simulink model "MainPlanevsRainCameras"  (R2020a)
(part 3 of 6)

  Radar3 : drivingscenarioandsensors/Radar Detection Generator  SensorIndex=5  UpdateInterval=0.1  SensorLocation=[0 0.9]  Height=0.2  Yaw=170.804327895794  Pitch=0  Roll=0  BusNameSource=Auto  BusName=BusRadarDetectionGenerator  MaxNumDetectionsSource=Property  MaxNumDetections=50  DetectionCoordinates=Ego Cartesian  SimulateUsing=Interpreted execution  AzimuthResolution=4  ElevationResolution=10  RangeResolution=2.5  RangeRateResolution=0.5  AzimuthBiasFraction=0.1  ElevationBiasFraction=0.1  RangeBiasFraction=0.05  RangeRateBiasFraction=0.05  FieldOfView=[90 2.5]  MaxRange=10  RangeRateLimits=[-100 100]  DetectionProbability=0.9  FalseAlarmRate=1e-06  ReferenceRange=15  ReferenceRCS=0  HasElevation=on  HasRangeRate=off  HasNoise=on  HasFalseAlarms=on  HasOcclusion=on  InitialSeedSource=Repeatable  InitialSeed=0  UsedSeed=0  ActorProfilesSource=MATLAB expression  ActorProfilesParameters=driving.internal.ActorProfilesRadarParameters  ActorProfilesExpression=[struct('ActorID',1,'ClassID',1,'Length',4.7,'Width',1.8,'Height',1.4,'OriginOffset',[-1.35 0 0],'MeshVertices',[3.7 -0.9 1.4;3.7 0.9 1.4;-1 0.9 1.4;-1 -0.9 1.4;3.7 -0.9 0;3.7 0.9 0;-1 0.9 0;-1 -0.9 0],'MeshFaces',[6 2 1;1 5 6;8 4 3;3 7 8;6 7 3;3 2 6;5 1 4;4 8 5;4 1 2;2 3 4;7 6 5;5 8 7],'RCSPattern',[10 10;10 10],'RCSAzimuthAngles',[-180 180],'RCSElevationAngles',[-90 90]); struct('ActorID',2,'ClassID',1,'Length',4.7,'Width',1.8,'Height',1.4,'OriginOffset',[-1.35 0 0],'MeshVertices',[3.7 -0.9 1.4;3.7 0.9 1.4;-1 0.9 1.4;-1 -0.9 1.4;3.7 -0.9 0;3.7 0.9 0;-1 0.9 0;-1 -0.9 0],'MeshFaces',[6 2 1;1 5 6;8 4 3;3 7 8;6 7 3;3 2 6;5 1 4;4 8 5;4 1 2;2 3 4;7 6 5;5 8 7],'RCSPattern',[10 10;10 10],'RCSAzimuthAngles',[-180 180],'RCSElevationAngles',[-90 90]); struct('ActorID',3,'ClassID',1,'Length',4.7,'Width',1.8,'Height',1.4,'OriginOffset',[-1.35 0 0],'MeshVertices',[3.7 -0.9 1.4;3.7 0.9 1.4;-1 0.9 1.4;-1 -0.9 1.4;3.7 -0.9 0;3.7 0.9 0;-1 0.9 0;-1 -0.9 0],'MeshFaces',[6 2 1;1 5 6;8 4 3;3 7 8;6 7 3;3 2 6;5 1 4;4 8 5;4 1 2;2 3 4;7 6 5;5 8 7],'RCSPattern',[10 10;10 10],'RCSAzimuthAngles',[-180 180],'RCSElevationAngles',[-90 90]); struct('ActorID',4,'ClassID',1,'Length',4.7,'Width',1.8,'Height',1.4,'OriginOffset',[-1.35 0 0],'MeshVertices',[3.7 -0.9 1.4;3.7 0.9 1.4;-1 0.9 1.4;-1 -0.9 1.4;3.7 -0.9 0;3.7 0.9 0;-1 0.9 0;-1 -0.9 0],'MeshFaces',[6 2 1;1 5 6;8 4 3;3 7 8;6 7 3;3 2 6;5 1 4;4 8 5;4 1 2;2 3 4;7 6 5;5 8 7],'RCSPattern',[10 10;10 10],'RCSAzimuthAngles',[-180 180],'RCSElevationAngles',[-90 90]); struct('ActorID',5,'ClassID',1,'Length',4.7,'Width',1.8,'Height',1.4,'OriginOffset',[-1.35 0 0],'MeshVertices',[3.7 -0.9 1.4;3.7 0.9 1.4;-1 0.9 1.4;-1 -0.9 1.4;3.7 -0.9 0;3.7 0.9 0;-1 0.9 0;-1 -0.9 0],'MeshFaces',[6 2 1;1 5 6;8 4 3;3 7 8;6 7 3;3 2 6;5 1 4;4 8 5;4 1 2;2 3 4;7 6 5;5 8 7],'RCSPattern',[10 10;10 10],'RCSAzimuthAngles',[-180 180],'RCSElevationAngles',[-90 90]); struct('ActorID',6,'ClassID',4,'Length',0.24,'Width',0.45,'Height',1.7,'OriginOffset',[0 0 0],'MeshVertices',[0.12 -0.225 1.7;0.12 0.225 1.7;-0.12 0.225 1.7;-0.12 -0.225 1.7;0.12 -0.225 -1.11022302462516e-16;0.12 0.225 -1.11022302462516e-16;-0.12 0.225 -1.11022302462516e-16;-0.12 -0.225 -1.11022302462516e-16],'MeshFaces',[6 2 1;1 5 6;8 4 3;3 7 8;6 7 3;3 2 6;5 1 4;4 8 5;4 1 2;2 3 4;7 6 5;5 8 7],'RCSPattern',[-8 -8;-8 -8],'RCSAzimuthAngles',[-180 180],'RCSElevationAngles',[-90 90]); struct('ActorID',7,'ClassID',4,'Length',0.24,'Width',0.45,'Height',1.7,'OriginOffset',[0 0 0],'MeshVertices',[0.12 -0.225 1.7;0.12 0.225 1.7;-0.12 0.225 1.7;-0.12 -0.225 1.7;0.12 -0.225 -1.11022302462516e-16;0.12 0.225 -1.11022302462516e-16;-0.12 0.225 -1.11022302462516e-16;-0.12 -0.225 -1.11022302462516e-16],'MeshFaces',[6 2 1;1 5 6;8 4 3;3 7 8;6 7 3;3 2 6;5 1 4;4 8 5;4 1 2;2 3 4;7 6 5;5 8 7],'RCSPattern',[-8 -8;-8 -8],'RCSAzimuthAngles',[-180 180],'RCSElevationAngles',[-90 90]); struct('ActorID',8,'ClassID',4,'Length',0.24,'Width',0.45,'Height',1.7,'OriginOffset',[0 0 0],'MeshVertices',[0.12 -0.225 1.7;0.12 0.225 1.7;-0.12 0.225 1.7;-0.12 -0.225 1.7;0.12 -0.225 -1.11022302462516e-16;0.12 0.225 -1.11022302462516e-16;-0.12 0.225 -1.11022302462516e-16;-0.12 -0.225 -1.11022302462516e-16],'MeshFaces',[6 2 1;1 5 6;8 4 3;3 7 8;6 7 3;3 2 6;5 1 4;4 8 5;4 1 2;2 3 4;7 6 5;5 8 7],'RCSPattern',[-8 -8;-8 -8],'RCSAzimuthAngles',[-180 180],'RCSElevationAngles',[-90 90]); struct('ActorID',9,'ClassID',4,'Length',0.24,'Width',0.45,'Height',1.7,'OriginOffset',[0 0 0],'MeshVertices',[0.12 -0.225 1.7;0.12 0.225 1.7;-0.12 0.225 1.7;-0.12 -0.225 1.7;0.12 -0.225 -1.11022302462516e-16;0.12 0.225 -1.11022302462516e-16;-0.12 0.225 -1.11022302462516e-16;-0.12 -0.225 -1.11022302462516e-16],'MeshFaces',[6 2 1;1 5 6;8 4 3;3 7 8;6 7 3;3 2 6;5 1 4;4 8 5;4 1 2;2 3 4;7 6 5;5 8 7],'RCSPattern',[-8 -8;-8 -8],'RCSAzimuthAngles',[-180 180],'RCSElevationAngles',[-90 90]); struct('ActorID',10,'ClassID',4,'Length',0.24,'Width',0.45,'Height',1.7,'OriginOffset',[0 0 0],'MeshVertices',[0.12 -0.225 1.7;0.12 0.225 1.7;-0.12 0.225 1.7;-0.12 -0.225 1.7;0.12 -0.225 -1.11022302462516e-16;0.12 0.225 -1.11022302462516e-16;-0.12 0.225 -1.11022302462516e-16;-0.12 -0.225 -1.11022302462516e-16],'MeshFaces',[6 2 1;1 5 6;8 4 3;3 7 8;6 7 3;3 2 6;5 1 4;4 8 5;4 1 2;2 3 4;7 6 5;5 8 7],'RCSPattern',[-8 -8;-8 -8],'RCSAzimuthAngles',[-180 180],'RCSElevationAngles',[-90 90]); struct('ActorID',11,'ClassID',4,'Length',0.24,'Width',0.45,'Height',1.7,'OriginOffset',[0 0 0],'MeshVertices',[0.12 -0.225 1.7;0.12 0.225 1.7;-0.12 0.225 1.7;-0.12 -0.225 1.7;0.12 -0.225 -1.11022302462516e-16;0.12 0.225 -1.11022302462516e-16;-0.12 0.225 -1.11022302462516e-16;-0.12 -0.225 -1.11022302462516e-16],'MeshFaces',[6 2 1;1 5 6;8 4 3;3 7 8;6 7 3;3 2 6;5 1 4;4 8 5;4 1 2;2 3 4;7 6 5;5 8 7],'RCSPattern',[-8 -8;-8 -8],'RCSAzimuthAngles',[-180 180],'RCSElevationAngles',[-90 90]); struct('ActorID',12,'ClassID',4,'Length',0.24,'Width',0.45,'Height',1.7,'OriginOffset',[0 0 0],'MeshVertices',[0.12 -0.225 1.7;0.12 0.225 1.7;-0.12 0.225 1.7;-0.12 -0.225 1.7;0.12 -0.225 -1.11022302462516e-16;0.12 0.225 -1.11022302462516e-16;-0.12 0.225 -1.11022302462516e-16;-0.12 -0.225 -1.11022302462516e-16],'MeshFaces',[6 2 1;1 5 6;8 4 3;3 7 8;6 7 3;3 2 6;5 1 4;4 8 5;4 1 2;2 3 4;7 6 5;5 8 7],'RCSPattern',[-8 -8;-8 -8],'RCSAzimuthAngles',[-180 180],'RCSElevationAngles',[-90 90]); struct('ActorID',13,'ClassID',4,'Length',0.24,'Width',0.45,'Height',1.7,'OriginOffset',[0 0 0],'MeshVertices',[0.12 -0.225 1.7;0.12 0.225 1.7;-0.12 0.225 1.7;-0.12 -0.225 1.7;0.12 -0.225 -1.11022302462516e-16;0.12 0.225 -1.11022302462516e-16;-0.12 0.225 -1.11022302462516e-16;-0.12 -0.225 -1.11022302462516e-16],'MeshFaces',[6 2 1;1 5 6;8 4 3;3 7 8;6 7 3;3 2 6;5 1 4;4 8 5;4 1 2;2 3 4;7 6 5;5 8 7],'RCSPattern',[-8 -8;-8 -8],'RCSAzimuthAngles',[-180 180],'RCSElevationAngles',[-90 90]); struct('ActorID',14,'ClassID',4,'Length',0.24,'Width',0.45,'Height',1.7,'OriginOffset',[0 0 0],'MeshVertices',[0.12 -0.225 1.7;0.12 0.225 1.7;-0.12 0.225 1.7;-0.12 -0.225 1.7;0.12 -0.225 -1.11022302462516e-16;0.12 0.225 -1.11022302462516e-16;-0.12 0.225 -1.11022302462516e-16;-0.12 -0.225 -1.11022302462516e-16],'MeshFaces',[6 2 1;1 5 6;8 4 3;3 7 8;6 7 3;3 2 6;5 1 4;4 8 5;4 1 2;2 3 4;7 6 5;5 8 7],'RCSPattern',[-8 -8;-8 -8],'RCSAzimuthAngles',[-180 180],'RCSElevationAngles',[-90 90]); struct('ActorID',15,'ClassID',4,'Length',0.24,'Width',0.45,'Height',1.7,'OriginOffset',[0 0 0],'MeshVertices',[0.12 -0.225 1.7;0.12 0.225 1.7;-0.12 0.225 1.7;-0.12 -0.225 1.7;0.12 -0.225 -1.11022302462516e-16;0.12 0.225 -1.11022302462516e-16;-0.12 0.225 -1.11022302462516e-16;-0.12 -0.225 -1.11022302462516e-16],'MeshFaces',[6 2 1;1 5 6;8 4 3;3 7 8;6 7 3;3 2 6;5 1 4;4 8 5;4 1 2;2 3 4;7 6 5;5 8 7],'RCSPattern',[-8 -8;-8 -8],'RCSAzimuthAngles',[-180 180],'RCSElevationAngles',[-90 90]); struct('ActorID',16,'ClassID',4,'Length',0.24,'Width',0.45,'Height',1.7,'OriginOffset',[0 0 0],'MeshVertices',[0.12 -0.225 1.7;0.12 0.225 1.7;-0.12 0.225 1.7;-0.12 -0.225 1.7;0.12 -0.225 -1.11022302462516e-16;0.12 0.225 -1.11022302462516e-16;-0.12 0.225 -1.11022302462516e-16;-0.12 -0.225 -1.11022302462516e-16],'MeshFaces',[6 2 1;1 5 6;8 4 3;3 7 8;6 7 3;3 2 6;5 1 4;4 8 5;4 1 2;2 3 4;7 6 5;5 8 7],'RCSPattern',[-8 -8;-8 -8],'RCSAzimuthAngles',[-180 180],'RCSElevationAngles',[-90 90]); struct('ActorID',17,'ClassID',4,'Length',0.24,'Width',0.45,'Height',1.7,'OriginOffset',[0 0 0],'MeshVertices',[0.12 -0.225 1.7;0.12 0.225 1.7;-0.12 0.225 1.7;-0.12 -0.225 1.7;0.12 -0.225 -1.11022302462516e-16;0.12 0.225 -1.11022302462516e-16;-0.12 0.225 -1.11022302462516e-16;-0.12 -0.225 -1.11022302462516e-16],'MeshFaces',[6 2 1;1 5 6;8 4 3;3 7 8;6 7 3;3 2 6;5 1 4;4 8 5;4 1 2;2 3 4;7 6 5;5 8 7],'RCSPattern',[-8 -8;-8 -8],'RCSAzimuthAngles',[-180 180],'RCSElevationAngles',[-90 90]); struct('ActorID',18,'ClassID',4,'Length',0.24,'Width',0.45,'Height',1.7,'OriginOffset',[0 0 0],'MeshVertices',[0.12 -0.225 1.7;0.12 0.225 1.7;-0.12 0.225 1.7;-0.12 -0.225 1.7;0.12 -0.225 -1.11022302462516e-16;0.12 0.225 -1.11022302462516e-16;-0.12 0.225 -1.11022302462516e-16;-0.12 -0.225 -1.11022302462516e-16],'MeshFaces',[6 2 1;1 5 6;8 4 3;3 7 8;6 7 3;3 2 6;5 1 4;4 8 5;4 1 2;2 3 4;7 6 5;5 8 7],'RCSPattern',[-8 -8;-8 -8],'RCSAzimuthAngles',[-180 180],'RCSElevationAngles',[-90 90]); struct('ActorID',19,'ClassID',4,'Length',0.24,'Width',0.45,'Height',1.7,'OriginOffset',[0 0 0],'MeshVertices',[0.12 -0.225 1.7;0.12 0.225 1.7;-0.12 0.225 1.7;-0.12 -0.225 1.7;0.12 -0.225 -1.11022302462516e-16;0.12 0.225 -1.11022302462516e-16;-0.12 0.225 -1.11022302462516e-16;-0.12 -0.225 -1.11022302462516e-16],'MeshFaces',[6 2 1;1 5 6;8 4 3;3 7 8;6 7 3;3 2 6;5 1 4;4 8 5;4 1 2;2 3 4;7 6 5;5 8 7],'RCSPattern',[-8 -8;-8 -8],'RCSAzimuthAngles',[-180 180],'RCSElevationAngles',[-90 90]); struct('ActorID',20,'ClassID',4,'Length',0.24,'Width',0.45,'Height',1.7,'OriginOffset',[0 0 0],'MeshVertices',[0.12 -0.225 1.7;0.12 0.225 1.7;-0.12 0.225 1.7;-0.12 -0.225 1.7;0.12 -0.225 -1.11022302462516e-16;0.12 0.225 -1.11022302462516e-16;-0.12 0.225 -1.11022302462516e-16;-0.12 -0.225 -1.11022302462516e-16],'MeshFaces',[6 2 1;1 5 6;8 4 3;3 7 8;6 7 3;3 2 6;5 1 4;4 8 5;4 1 2;2 3 4;7 6 5;5 8 7],'RCSPattern',[-8 -8;-8 -8],'RCSAzimuthAngles',[-180 180],'RCSElevationAngles',[-90 90]); struct('ActorID',21,'ClassID',4,'Length',0.24,'Width',0.45,'Height',1.7,'OriginOffset',[0 0 0],'MeshVertices',[0.12 -0.225 1.7;0.12 0.225 1.7;-0.12 0.225 1.7;-0.12 -0.225 1.7;0.12 -0.225 -1.11022302462516e-16;0.12 0.225 -1.11022302462516e-16;-0.12 0.225 -1.11022302462516e-16;-0.12 -0.225 -1.11022302462516e-16],'MeshFaces',[6 2 1;1 5 6;8 4 3;3 7 8;6 7 3;3 2 6;5 1 4;4 8 5;4 1 2;2 3 4;7 6 5;5 8 7],'RCSPattern',[-8 -8;-8 -8],'RCSAzimuthAngles',[-180 180],'RCSElevationAngles',[-90 90]); struct('ActorID',22,'ClassID',4,'Length',0.24,'Width',0.45,'Height',1.7,'OriginOffset',[0 0 0],'MeshVertices',[0.12 -0.225 1.7;0.12 0.225 1.7;-0.12 0.225 1.7;-0.12 -0.225 1.7;0.12 -0.225 -1.11022302462516e-16;0.12 0.225 -1.11022302462516e-16;-0.12 0.225 -1.11022302462516e-16;-0.12 -0.225 -1.11022302462516e-16],'MeshFaces',[6 2 1;1 5 6;8 4 3;3 7 8;6 7 3;3 2 6;5 1 4;4 8 5;4 1 2;2 3 4;7 6 5;5 8 7],'RCSPattern',[-8 -8;-8 -8],'RCSAzimuthAngles',[-180 180],'RCSElevationAngles',[-90 90]); struct('ActorID',23,'ClassID',4,'Length',0.24,'Width',0.45,'Height',1.7,'OriginOffset',[0 0 0],'MeshVertices',[0.12 -0.225 1.7;0.12 0.225 1.7;-0.12 0.225 1.7;-0.12 -0.225 1.7;0.12 -0.225 -1.11022302462516e-16;0.12 0.225 -1.11022302462516e-16;-0.12 0.225 -1.11022302462516e-16;-0.12 -0.225 -1.11022302462516e-16],'MeshFaces',[6 2 1;1 5 6;8 4 3;3 7 8;6 7 3;3 2 6;5 1 4;4 8 5;4 1 2;2 3 4;7 6 5;5 8 7],'RCSPattern',[-8 -8;-8 -8],'RCSAzimuthAngles',[-180 180],'RCSElevationAngles',[-90 90]); struct('ActorID',24,'ClassID',4,'Length',0.24,'Width',0.45,'Height',1.7,'OriginOffset',[0 0 0],'MeshVertices',[0.12 -0.225 1.7;0.12 0.225 1.7;-0.12 0.225 1.7;-0.12 -0.225 1.7;0.12 -0.225 -1.11022302462516e-16;0.12 0.225 -1.11022302462516e-16;-0.12 0.225 -1.11022302462516e-16;-0.12 -0.225 -1.11022302462516e-16],'MeshFaces',[6 2 1;1 5 6;8 4 3;3 7 8;6 7 3;3 2 6;5 1 4;4 8 5;4 1 2;2 3 4;7 6 5;5 8 7],'RCSPattern',[-8 -8;-8 -8],'RCSAzimuthAngles',[-180 180],'RCSElevationAngles',[-90 90]); struct('ActorID',25,'ClassID',4,'Length',0.24,'Width',0.45,'Height',1.7,'OriginOffset',[0 0 0],'MeshVertices',[0.12 -0.225 1.7;0.12 0.225 1.7;-0.12 0.225 1.7;-0.12 -0.225 1.7;0.12 -0.225 -1.11022302462516e-16;0.12 0.225 -1.11022302462516e-16;-0.12 0.225 -1.11022302462516e-16;-0.12 -0.225 -1.11022302462516e-16],'MeshFaces',[6 2 1;1 5 6;8 4 3;3 7 8;6 7 3;3 2 6;5 1 4;4 8 5;4 1 2;2 3 4;7 6 5;5 8 7],'RCSPattern',[-8 -8;-8 -8],'RCSAzimuthAngles',[-180 180],'RCSElevationAngles',[-90 90]); struct('ActorID',26,'ClassID',4,'Length',0.24,'Width',0.45,'Height',1.7,'OriginOffset',[0 0 0],'MeshVertices',[0.12 -0.225 1.7;0.12 0.225 1.7;-0.12 0.225 1.7;-0.12 -0.225 1.7;0.12 -0.225 -1.11022302462516e-16;0.12 0.225 -1.11022302462516e-16;-0.12 0.225 -1.11022302462516e-16;-0.12 -0.225 -1.11022302462516e-16],'MeshFaces',[6 2 1;1 5 6;8 4 3;3 7 8;6 7 3;3 2 6;5 1 4;4 8 5;4 1 2;2 3 4;7 6 5;5 8 7],'RCSPattern',[-8 -8;-8 -8],'RCSAzimuthAngles',[-180 180],'RCSElevationAngles',[-90 90]); struct('ActorID',27,'ClassID',4,'Length',0.24,'Width',0.45,'Height',1.7,'OriginOffset',[0 0 0],'MeshVertices',[0.12 -0.225 1.7;0.12 0.225 1.7;-0.12 0.225 1.7;-0.12 -0.225 1.7;0.12 -0.225 -1.11022302462516e-16;0.12 0.225 -1.11022302462516e-16;-0.12 0.225 -1.11022302462516e-16;-0.12 -0.225 -1.11022302462516e-16],'MeshFaces',[6 2 1;1 5 6;8 4 3;3 7 8;6 7 3;3 2 6;5 1 4;4 8 5;4 1 2;2 3 4;7 6 5;5 8 7],'RCSPattern',[-8 -8;-8 -8],'RCSAzimuthAngles',[-180 180],'RCSElevationAngles',[-90 90]); struct('ActorID',28,'ClassID',3,'Length',1.7,'Width',0.45,'Height',1.7,'OriginOffset',[0 0 0],'MeshVertices',[0.85 -0.225 1.7;0.85 0.225 1.7;-0.85 0.225 1.7;-0.85 -0.225 1.7;0.85 -0.225 -1.11022302462516e-16;0.85 0.225 -1.11022302462516e-16;-0.85 0.225 -1.11022302462516e-16;-0.85 -0.225 -1.11022302462516e-16],'MeshFaces',[6 2 1;1 5 6;8 4 3;3 7 8;6 7 3;3 2 6;5 1 4;4 8 5;4 1 2;2 3 4;7 6 5;5 8 7],'RCSPattern',[10 10;10 10],'RCSAzimuthAngles',[-180 180],'RCSElevationAngles',[-90 90]); struct('ActorID',29,'ClassID',4,'Length',0.24,'Width',0.45,'Height',1.7,'OriginOffset',[0 0 0],'MeshVertices',[0.12 -0.225 1.7;0.12 0.225 1.7;-0.12 0.225 1.7;-0.12 -0.225 1.7;0.12 -0.225 -1.11022302462516e-16;0.12 0.225 -1.11022302462516e-16;-0.12 0.225 -1.11022302462516e-16;-0.12 -0.225 -1.11022302462516e-16],'MeshFaces',[6 2 1;1 5 6;8 4 3;3 7 8;6 7 3;3 2 6;5 1 4;4 8 5;4 1 2;2 3 4;7 6 5;5 8 7],'RCSPattern',[-8 -8;-8 -8],'RCSAzimuthAngles',[-180 180],'RCSElevationAngles',[-90 90])]
      settings: SourceProductBaseCode=DR
  Radar4 : drivingscenarioandsensors/Radar Detection Generator  SensorIndex=6  UpdateInterval=0.1  SensorLocation=[0 -0.9]  Height=0.2  Yaw=-171.21089543369  Pitch=0  Roll=0  BusNameSource=Auto  BusName=BusRadarDetectionGenerator  MaxNumDetectionsSource=Property  MaxNumDetections=50  DetectionCoordinates=Ego Cartesian  SimulateUsing=Interpreted execution  AzimuthResolution=4  ElevationResolution=10  RangeResolution=2.5  RangeRateResolution=0.5  AzimuthBiasFraction=0.1  ElevationBiasFraction=0.1  RangeBiasFraction=0.05  RangeRateBiasFraction=0.05  FieldOfView=[90 2.5]  MaxRange=10  RangeRateLimits=[-100 100]  DetectionProbability=0.9  FalseAlarmRate=1e-06  ReferenceRange=15  ReferenceRCS=0  HasElevation=on  HasRangeRate=off  HasNoise=on  HasFalseAlarms=on  HasOcclusion=on  InitialSeedSource=Repeatable  InitialSeed=0  UsedSeed=0  ActorProfilesSource=MATLAB expression  ActorProfilesParameters=driving.internal.ActorProfilesRadarParameters  ActorProfilesExpression=[struct('ActorID',1,'ClassID',1,'Length',4.7,'Width',1.8,'Height',1.4,'OriginOffset',[-1.35 0 0],'MeshVertices',[3.7 -0.9 1.4;3.7 0.9 1.4;-1 0.9 1.4;-1 -0.9 1.4;3.7 -0.9 0;3.7 0.9 0;-1 0.9 0;-1 -0.9 0],'MeshFaces',[6 2 1;1 5 6;8 4 3;3 7 8;6 7 3;3 2 6;5 1 4;4 8 5;4 1 2;2 3 4;7 6 5;5 8 7],'RCSPattern',[10 10;10 10],'RCSAzimuthAngles',[-180 180],'RCSElevationAngles',[-90 90]); struct('ActorID',2,'ClassID',1,'Length',4.7,'Width',1.8,'Height',1.4,'OriginOffset',[-1.35 0 0],'MeshVertices',[3.7 -0.9 1.4;3.7 0.9 1.4;-1 0.9 1.4;-1 -0.9 1.4;3.7 -0.9 0;3.7 0.9 0;-1 0.9 0;-1 -0.9 0],'MeshFaces',[6 2 1;1 5 6;8 4 3;3 7 8;6 7 3;3 2 6;5 1 4;4 8 5;4 1 2;2 3 4;7 6 5;5 8 7],'RCSPattern',[10 10;10 10],'RCSAzimuthAngles',[-180 180],'RCSElevationAngles',[-90 90]); struct('ActorID',3,'ClassID',1,'Length',4.7,'Width',1.8,'Height',1.4,'OriginOffset',[-1.35 0 0],'MeshVertices',[3.7 -0.9 1.4;3.7 0.9 1.4;-1 0.9 1.4;-1 -0.9 1.4;3.7 -0.9 0;3.7 0.9 0;-1 0.9 0;-1 -0.9 0],'MeshFaces',[6 2 1;1 5 6;8 4 3;3 7 8;6 7 3;3 2 6;5 1 4;4 8 5;4 1 2;2 3 4;7 6 5;5 8 7],'RCSPattern',[10 10;10 10],'RCSAzimuthAngles',[-180 180],'RCSElevationAngles',[-90 90]); struct('ActorID',4,'ClassID',1,'Length',4.7,'Width',1.8,'Height',1.4,'OriginOffset',[-1.35 0 0],'MeshVertices',[3.7 -0.9 1.4;3.7 0.9 1.4;-1 0.9 1.4;-1 -0.9 1.4;3.7 -0.9 0;3.7 0.9 0;-1 0.9 0;-1 -0.9 0],'MeshFaces',[6 2 1;1 5 6;8 4 3;3 7 8;6 7 3;3 2 6;5 1 4;4 8 5;4 1 2;2 3 4;7 6 5;5 8 7],'RCSPattern',[10 10;10 10],'RCSAzimuthAngles',[-180 180],'RCSElevationAngles',[-90 90]); struct('ActorID',5,'ClassID',1,'Length',4.7,'Width',1.8,'Height',1.4,'OriginOffset',[-1.35 0 0],'MeshVertices',[3.7 -0.9 1.4;3.7 0.9 1.4;-1 0.9 1.4;-1 -0.9 1.4;3.7 -0.9 0;3.7 0.9 0;-1 0.9 0;-1 -0.9 0],'MeshFaces',[6 2 1;1 5 6;8 4 3;3 7 8;6 7 3;3 2 6;5 1 4;4 8 5;4 1 2;2 3 4;7 6 5;5 8 7],'RCSPattern',[10 10;10 10],'RCSAzimuthAngles',[-180 180],'RCSElevationAngles',[-90 90]); struct('ActorID',6,'ClassID',4,'Length',0.24,'Width',0.45,'Height',1.7,'OriginOffset',[0 0 0],'MeshVertices',[0.12 -0.225 1.7;0.12 0.225 1.7;-0.12 0.225 1.7;-0.12 -0.225 1.7;0.12 -0.225 -1.11022302462516e-16;0.12 0.225 -1.11022302462516e-16;-0.12 0.225 -1.11022302462516e-16;-0.12 -0.225 -1.11022302462516e-16],'MeshFaces',[6 2 1;1 5 6;8 4 3;3 7 8;6 7 3;3 2 6;5 1 4;4 8 5;4 1 2;2 3 4;7 6 5;5 8 7],'RCSPattern',[-8 -8;-8 -8],'RCSAzimuthAngles',[-180 180],'RCSElevationAngles',[-90 90]); struct('ActorID',7,'ClassID',4,'Length',0.24,'Width',0.45,'Height',1.7,'OriginOffset',[0 0 0],'MeshVertices',[0.12 -0.225 1.7;0.12 0.225 1.7;-0.12 0.225 1.7;-0.12 -0.225 1.7;0.12 -0.225 -1.11022302462516e-16;0.12 0.225 -1.11022302462516e-16;-0.12 0.225 -1.11022302462516e-16;-0.12 -0.225 -1.11022302462516e-16],'MeshFaces',[6 2 1;1 5 6;8 4 3;3 7 8;6 7 3;3 2 6;5 1 4;4 8 5;4 1 2;2 3 4;7 6 5;5 8 7],'RCSPattern',[-8 -8;-8 -8],'RCSAzimuthAngles',[-180 180],'RCSElevationAngles',[-90 90]); struct('ActorID',8,'ClassID',4,'Length',0.24,'Width',0.45,'Height',1.7,'OriginOffset',[0 0 0],'MeshVertices',[0.12 -0.225 1.7;0.12 0.225 1.7;-0.12 0.225 1.7;-0.12 -0.225 1.7;0.12 -0.225 -1.11022302462516e-16;0.12 0.225 -1.11022302462516e-16;-0.12 0.225 -1.11022302462516e-16;-0.12 -0.225 -1.11022302462516e-16],'MeshFaces',[6 2 1;1 5 6;8 4 3;3 7 8;6 7 3;3 2 6;5 1 4;4 8 5;4 1 2;2 3 4;7 6 5;5 8 7],'RCSPattern',[-8 -8;-8 -8],'RCSAzimuthAngles',[-180 180],'RCSElevationAngles',[-90 90]); struct('ActorID',9,'ClassID',4,'Length',0.24,'Width',0.45,'Height',1.7,'OriginOffset',[0 0 0],'MeshVertices',[0.12 -0.225 1.7;0.12 0.225 1.7;-0.12 0.225 1.7;-0.12 -0.225 1.7;0.12 -0.225 -1.11022302462516e-16;0.12 0.225 -1.11022302462516e-16;-0.12 0.225 -1.11022302462516e-16;-0.12 -0.225 -1.11022302462516e-16],'MeshFaces',[6 2 1;1 5 6;8 4 3;3 7 8;6 7 3;3 2 6;5 1 4;4 8 5;4 1 2;2 3 4;7 6 5;5 8 7],'RCSPattern',[-8 -8;-8 -8],'RCSAzimuthAngles',[-180 180],'RCSElevationAngles',[-90 90]); struct('ActorID',10,'ClassID',4,'Length',0.24,'Width',0.45,'Height',1.7,'OriginOffset',[0 0 0],'MeshVertices',[0.12 -0.225 1.7;0.12 0.225 1.7;-0.12 0.225 1.7;-0.12 -0.225 1.7;0.12 -0.225 -1.11022302462516e-16;0.12 0.225 -1.11022302462516e-16;-0.12 0.225 -1.11022302462516e-16;-0.12 -0.225 -1.11022302462516e-16],'MeshFaces',[6 2 1;1 5 6;8 4 3;3 7 8;6 7 3;3 2 6;5 1 4;4 8 5;4 1 2;2 3 4;7 6 5;5 8 7],'RCSPattern',[-8 -8;-8 -8],'RCSAzimuthAngles',[-180 180],'RCSElevationAngles',[-90 90]); struct('ActorID',11,'ClassID',4,'Length',0.24,'Width',0.45,'Height',1.7,'OriginOffset',[0 0 0],'MeshVertices',[0.12 -0.225 1.7;0.12 0.225 1.7;-0.12 0.225 1.7;-0.12 -0.225 1.7;0.12 -0.225 -1.11022302462516e-16;0.12 0.225 -1.11022302462516e-16;-0.12 0.225 -1.11022302462516e-16;-0.12 -0.225 -1.11022302462516e-16],'MeshFaces',[6 2 1;1 5 6;8 4 3;3 7 8;6 7 3;3 2 6;5 1 4;4 8 5;4 1 2;2 3 4;7 6 5;5 8 7],'RCSPattern',[-8 -8;-8 -8],'RCSAzimuthAngles',[-180 180],'RCSElevationAngles',[-90 90]); struct('ActorID',12,'ClassID',4,'Length',0.24,'Width',0.45,'Height',1.7,'OriginOffset',[0 0 0],'MeshVertices',[0.12 -0.225 1.7;0.12 0.225 1.7;-0.12 0.225 1.7;-0.12 -0.225 1.7;0.12 -0.225 -1.11022302462516e-16;0.12 0.225 -1.11022302462516e-16;-0.12 0.225 -1.11022302462516e-16;-0.12 -0.225 -1.11022302462516e-16],'MeshFaces',[6 2 1;1 5 6;8 4 3;3 7 8;6 7 3;3 2 6;5 1 4;4 8 5;4 1 2;2 3 4;7 6 5;5 8 7],'RCSPattern',[-8 -8;-8 -8],'RCSAzimuthAngles',[-180 180],'RCSElevationAngles',[-90 90]); struct('ActorID',13,'ClassID',4,'Length',0.24,'Width',0.45,'Height',1.7,'OriginOffset',[0 0 0],'MeshVertices',[0.12 -0.225 1.7;0.12 0.225 1.7;-0.12 0.225 1.7;-0.12 -0.225 1.7;0.12 -0.225 -1.11022302462516e-16;0.12 0.225 -1.11022302462516e-16;-0.12 0.225 -1.11022302462516e-16;-0.12 -0.225 -1.11022302462516e-16],'MeshFaces',[6 2 1;1 5 6;8 4 3;3 7 8;6 7 3;3 2 6;5 1 4;4 8 5;4 1 2;2 3 4;7 6 5;5 8 7],'RCSPattern',[-8 -8;-8 -8],'RCSAzimuthAngles',[-180 180],'RCSElevationAngles',[-90 90]); struct('ActorID',14,'ClassID',4,'Length',0.24,'Width',0.45,'Height',1.7,'OriginOffset',[0 0 0],'MeshVertices',[0.12 -0.225 1.7;0.12 0.225 1.7;-0.12 0.225 1.7;-0.12 -0.225 1.7;0.12 -0.225 -1.11022302462516e-16;0.12 0.225 -1.11022302462516e-16;-0.12 0.225 -1.11022302462516e-16;-0.12 -0.225 -1.11022302462516e-16],'MeshFaces',[6 2 1;1 5 6;8 4 3;3 7 8;6 7 3;3 2 6;5 1 4;4 8 5;4 1 2;2 3 4;7 6 5;5 8 7],'RCSPattern',[-8 -8;-8 -8],'RCSAzimuthAngles',[-180 180],'RCSElevationAngles',[-90 90]); struct('ActorID',15,'ClassID',4,'Length',0.24,'Width',0.45,'Height',1.7,'OriginOffset',[0 0 0],'MeshVertices',[0.12 -0.225 1.7;0.12 0.225 1.7;-0.12 0.225 1.7;-0.12 -0.225 1.7;0.12 -0.225 -1.11022302462516e-16;0.12 0.225 -1.11022302462516e-16;-0.12 0.225 -1.11022302462516e-16;-0.12 -0.225 -1.11022302462516e-16],'MeshFaces',[6 2 1;1 5 6;8 4 3;3 7 8;6 7 3;3 2 6;5 1 4;4 8 5;4 1 2;2 3 4;7 6 5;5 8 7],'RCSPattern',[-8 -8;-8 -8],'RCSAzimuthAngles',[-180 180],'RCSElevationAngles',[-90 90]); struct('ActorID',16,'ClassID',4,'Length',0.24,'Width',0.45,'Height',1.7,'OriginOffset',[0 0 0],'MeshVertices',[0.12 -0.225 1.7;0.12 0.225 1.7;-0.12 0.225 1.7;-0.12 -0.225 1.7;0.12 -0.225 -1.11022302462516e-16;0.12 0.225 -1.11022302462516e-16;-0.12 0.225 -1.11022302462516e-16;-0.12 -0.225 -1.11022302462516e-16],'MeshFaces',[6 2 1;1 5 6;8 4 3;3 7 8;6 7 3;3 2 6;5 1 4;4 8 5;4 1 2;2 3 4;7 6 5;5 8 7],'RCSPattern',[-8 -8;-8 -8],'RCSAzimuthAngles',[-180 180],'RCSElevationAngles',[-90 90]); struct('ActorID',17,'ClassID',4,'Length',0.24,'Width',0.45,'Height',1.7,'OriginOffset',[0 0 0],'MeshVertices',[0.12 -0.225 1.7;0.12 0.225 1.7;-0.12 0.225 1.7;-0.12 -0.225 1.7;0.12 -0.225 -1.11022302462516e-16;0.12 0.225 -1.11022302462516e-16;-0.12 0.225 -1.11022302462516e-16;-0.12 -0.225 -1.11022302462516e-16],'MeshFaces',[6 2 1;1 5 6;8 4 3;3 7 8;6 7 3;3 2 6;5 1 4;4 8 5;4 1 2;2 3 4;7 6 5;5 8 7],'RCSPattern',[-8 -8;-8 -8],'RCSAzimuthAngles',[-180 180],'RCSElevationAngles',[-90 90]); struct('ActorID',18,'ClassID',4,'Length',0.24,'Width',0.45,'Height',1.7,'OriginOffset',[0 0 0],'MeshVertices',[0.12 -0.225 1.7;0.12 0.225 1.7;-0.12 0.225 1.7;-0.12 -0.225 1.7;0.12 -0.225 -1.11022302462516e-16;0.12 0.225 -1.11022302462516e-16;-0.12 0.225 -1.11022302462516e-16;-0.12 -0.225 -1.11022302462516e-16],'MeshFaces',[6 2 1;1 5 6;8 4 3;3 7 8;6 7 3;3 2 6;5 1 4;4 8 5;4 1 2;2 3 4;7 6 5;5 8 7],'RCSPattern',[-8 -8;-8 -8],'RCSAzimuthAngles',[-180 180],'RCSElevationAngles',[-90 90]); struct('ActorID',19,'ClassID',4,'Length',0.24,'Width',0.45,'Height',1.7,'OriginOffset',[0 0 0],'MeshVertices',[0.12 -0.225 1.7;0.12 0.225 1.7;-0.12 0.225 1.7;-0.12 -0.225 1.7;0.12 -0.225 -1.11022302462516e-16;0.12 0.225 -1.11022302462516e-16;-0.12 0.225 -1.11022302462516e-16;-0.12 -0.225 -1.11022302462516e-16],'MeshFaces',[6 2 1;1 5 6;8 4 3;3 7 8;6 7 3;3 2 6;5 1 4;4 8 5;4 1 2;2 3 4;7 6 5;5 8 7],'RCSPattern',[-8 -8;-8 -8],'RCSAzimuthAngles',[-180 180],'RCSElevationAngles',[-90 90]); struct('ActorID',20,'ClassID',4,'Length',0.24,'Width',0.45,'Height',1.7,'OriginOffset',[0 0 0],'MeshVertices',[0.12 -0.225 1.7;0.12 0.225 1.7;-0.12 0.225 1.7;-0.12 -0.225 1.7;0.12 -0.225 -1.11022302462516e-16;0.12 0.225 -1.11022302462516e-16;-0.12 0.225 -1.11022302462516e-16;-0.12 -0.225 -1.11022302462516e-16],'MeshFaces',[6 2 1;1 5 6;8 4 3;3 7 8;6 7 3;3 2 6;5 1 4;4 8 5;4 1 2;2 3 4;7 6 5;5 8 7],'RCSPattern',[-8 -8;-8 -8],'RCSAzimuthAngles',[-180 180],'RCSElevationAngles',[-90 90]); struct('ActorID',21,'ClassID',4,'Length',0.24,'Width',0.45,'Height',1.7,'OriginOffset',[0 0 0],'MeshVertices',[0.12 -0.225 1.7;0.12 0.225 1.7;-0.12 0.225 1.7;-0.12 -0.225 1.7;0.12 -0.225 -1.11022302462516e-16;0.12 0.225 -1.11022302462516e-16;-0.12 0.225 -1.11022302462516e-16;-0.12 -0.225 -1.11022302462516e-16],'MeshFaces',[6 2 1;1 5 6;8 4 3;3 7 8;6 7 3;3 2 6;5 1 4;4 8 5;4 1 2;2 3 4;7 6 5;5 8 7],'RCSPattern',[-8 -8;-8 -8],'RCSAzimuthAngles',[-180 180],'RCSElevationAngles',[-90 90]); struct('ActorID',22,'ClassID',4,'Length',0.24,'Width',0.45,'Height',1.7,'OriginOffset',[0 0 0],'MeshVertices',[0.12 -0.225 1.7;0.12 0.225 1.7;-0.12 0.225 1.7;-0.12 -0.225 1.7;0.12 -0.225 -1.11022302462516e-16;0.12 0.225 -1.11022302462516e-16;-0.12 0.225 -1.11022302462516e-16;-0.12 -0.225 -1.11022302462516e-16],'MeshFaces',[6 2 1;1 5 6;8 4 3;3 7 8;6 7 3;3 2 6;5 1 4;4 8 5;4 1 2;2 3 4;7 6 5;5 8 7],'RCSPattern',[-8 -8;-8 -8],'RCSAzimuthAngles',[-180 180],'RCSElevationAngles',[-90 90]); struct('ActorID',23,'ClassID',4,'Length',0.24,'Width',0.45,'Height',1.7,'OriginOffset',[0 0 0],'MeshVertices',[0.12 -0.225 1.7;0.12 0.225 1.7;-0.12 0.225 1.7;-0.12 -0.225 1.7;0.12 -0.225 -1.11022302462516e-16;0.12 0.225 -1.11022302462516e-16;-0.12 0.225 -1.11022302462516e-16;-0.12 -0.225 -1.11022302462516e-16],'MeshFaces',[6 2 1;1 5 6;8 4 3;3 7 8;6 7 3;3 2 6;5 1 4;4 8 5;4 1 2;2 3 4;7 6 5;5 8 7],'RCSPattern',[-8 -8;-8 -8],'RCSAzimuthAngles',[-180 180],'RCSElevationAngles',[-90 90]); struct('ActorID',24,'ClassID',4,'Length',0.24,'Width',0.45,'Height',1.7,'OriginOffset',[0 0 0],'MeshVertices',[0.12 -0.225 1.7;0.12 0.225 1.7;-0.12 0.225 1.7;-0.12 -0.225 1.7;0.12 -0.225 -1.11022302462516e-16;0.12 0.225 -1.11022302462516e-16;-0.12 0.225 -1.11022302462516e-16;-0.12 -0.225 -1.11022302462516e-16],'MeshFaces',[6 2 1;1 5 6;8 4 3;3 7 8;6 7 3;3 2 6;5 1 4;4 8 5;4 1 2;2 3 4;7 6 5;5 8 7],'RCSPattern',[-8 -8;-8 -8],'RCSAzimuthAngles',[-180 180],'RCSElevationAngles',[-90 90]); struct('ActorID',25,'ClassID',4,'Length',0.24,'Width',0.45,'Height',1.7,'OriginOffset',[0 0 0],'MeshVertices',[0.12 -0.225 1.7;0.12 0.225 1.7;-0.12 0.225 1.7;-0.12 -0.225 1.7;0.12 -0.225 -1.11022302462516e-16;0.12 0.225 -1.11022302462516e-16;-0.12 0.225 -1.11022302462516e-16;-0.12 -0.225 -1.11022302462516e-16],'MeshFaces',[6 2 1;1 5 6;8 4 3;3 7 8;6 7 3;3 2 6;5 1 4;4 8 5;4 1 2;2 3 4;7 6 5;5 8 7],'RCSPattern',[-8 -8;-8 -8],'RCSAzimuthAngles',[-180 180],'RCSElevationAngles',[-90 90]); struct('ActorID',26,'ClassID',4,'Length',0.24,'Width',0.45,'Height',1.7,'OriginOffset',[0 0 0],'MeshVertices',[0.12 -0.225 1.7;0.12 0.225 1.7;-0.12 0.225 1.7;-0.12 -0.225 1.7;0.12 -0.225 -1.11022302462516e-16;0.12 0.225 -1.11022302462516e-16;-0.12 0.225 -1.11022302462516e-16;-0.12 -0.225 -1.11022302462516e-16],'MeshFaces',[6 2 1;1 5 6;8 4 3;3 7 8;6 7 3;3 2 6;5 1 4;4 8 5;4 1 2;2 3 4;7 6 5;5 8 7],'RCSPattern',[-8 -8;-8 -8],'RCSAzimuthAngles',[-180 180],'RCSElevationAngles',[-90 90]); struct('ActorID',27,'ClassID',4,'Length',0.24,'Width',0.45,'Height',1.7,'OriginOffset',[0 0 0],'MeshVertices',[0.12 -0.225 1.7;0.12 0.225 1.7;-0.12 0.225 1.7;-0.12 -0.225 1.7;0.12 -0.225 -1.11022302462516e-16;0.12 0.225 -1.11022302462516e-16;-0.12 0.225 -1.11022302462516e-16;-0.12 -0.225 -1.11022302462516e-16],'MeshFaces',[6 2 1;1 5 6;8 4 3;3 7 8;6 7 3;3 2 6;5 1 4;4 8 5;4 1 2;2 3 4;7 6 5;5 8 7],'RCSPattern',[-8 -8;-8 -8],'RCSAzimuthAngles',[-180 180],'RCSElevationAngles',[-90 90]); struct('ActorID',28,'ClassID',3,'Length',1.7,'Width',0.45,'Height',1.7,'OriginOffset',[0 0 0],'MeshVertices',[0.85 -0.225 1.7;0.85 0.225 1.7;-0.85 0.225 1.7;-0.85 -0.225 1.7;0.85 -0.225 -1.11022302462516e-16;0.85 0.225 -1.11022302462516e-16;-0.85 0.225 -1.11022302462516e-16;-0.85 -0.225 -1.11022302462516e-16],'MeshFaces',[6 2 1;1 5 6;8 4 3;3 7 8;6 7 3;3 2 6;5 1 4;4 8 5;4 1 2;2 3 4;7 6 5;5 8 7],'RCSPattern',[10 10;10 10],'RCSAzimuthAngles',[-180 180],'RCSElevationAngles',[-90 90]); struct('ActorID',29,'ClassID',4,'Length',0.24,'Width',0.45,'Height',1.7,'OriginOffset',[0 0 0],'MeshVertices',[0.12 -0.225 1.7;0.12 0.225 1.7;-0.12 0.225 1.7;-0.12 -0.225 1.7;0.12 -0.225 -1.11022302462516e-16;0.12 0.225 -1.11022302462516e-16;-0.12 0.225 -1.11022302462516e-16;-0.12 -0.225 -1.11022302462516e-16],'MeshFaces',[6 2 1;1 5 6;8 4 3;3 7 8;6 7 3;3 2 6;5 1 4;4 8 5;4 1 2;2 3 4;7 6 5;5 8 7],'RCSPattern',[-8 -8;-8 -8],'RCSAzimuthAngles',[-180 180],'RCSElevationAngles',[-90 90])]
      settings: SourceProductBaseCode=DR
  Radar5 : drivingscenarioandsensors/Radar Detection Generator  SensorIndex=12  UpdateInterval=0.1  SensorLocation=[1.9 0]  Height=0.2  Yaw=97.0523060078412  Pitch=0  Roll=0  BusNameSource=Auto  BusName=BusRadarDetectionGenerator  MaxNumDetectionsSource=Property  MaxNumDetections=50  DetectionCoordinates=Ego Cartesian  SimulateUsing=Interpreted execution  AzimuthResolution=4  ElevationResolution=10  RangeResolution=2.5  RangeRateResolution=0.5  AzimuthBiasFraction=0.1  ElevationBiasFraction=0.1  RangeBiasFraction=0.05  RangeRateBiasFraction=0.05  FieldOfView=[90 2.5]  MaxRange=10  RangeRateLimits=[-100 100]  DetectionProbability=0.9  FalseAlarmRate=1e-06  ReferenceRange=15  ReferenceRCS=0  HasElevation=on  HasRangeRate=off  HasNoise=on  HasFalseAlarms=on  HasOcclusion=on  InitialSeedSource=Repeatable  InitialSeed=0  UsedSeed=0  ActorProfilesSource=MATLAB expression  ActorProfilesParameters=driving.internal.ActorProfilesRadarParameters  ActorProfilesExpression=[struct('ActorID',1,'ClassID',1,'Length',4.7,'Width',1.8,'Height',1.4,'OriginOffset',[-1.35 0 0],'MeshVertices',[3.7 -0.9 1.4;3.7 0.9 1.4;-1 0.9 1.4;-1 -0.9 1.4;3.7 -0.9 0;3.7 0.9 0;-1 0.9 0;-1 -0.9 0],'MeshFaces',[6 2 1;1 5 6;8 4 3;3 7 8;6 7 3;3 2 6;5 1 4;4 8 5;4 1 2;2 3 4;7 6 5;5 8 7],'RCSPattern',[10 10;10 10],'RCSAzimuthAngles',[-180 180],'RCSElevationAngles',[-90 90]); struct('ActorID',2,'ClassID',1,'Length',4.7,'Width',1.8,'Height',1.4,'OriginOffset',[-1.35 0 0],'MeshVertices',[3.7 -0.9 1.4;3.7 0.9 1.4;-1 0.9 1.4;-1 -0.9 1.4;3.7 -0.9 0;3.7 0.9 0;-1 0.9 0;-1 -0.9 0],'MeshFaces',[6 2 1;1 5 6;8 4 3;3 7 8;6 7 3;3 2 6;5 1 4;4 8 5;4 1 2;2 3 4;7 6 5;5 8 7],'RCSPattern',[10 10;10 10],'RCSAzimuthAngles',[-180 180],'RCSElevationAngles',[-90 90]); struct('ActorID',3,'ClassID',1,'Length',4.7,'Width',1.8,'Height',1.4,'OriginOffset',[-1.35 0 0],'MeshVertices',[3.7 -0.9 1.4;3.7 0.9 1.4;-1 0.9 1.4;-1 -0.9 1.4;3.7 -0.9 0;3.7 0.9 0;-1 0.9 0;-1 -0.9 0],'MeshFaces',[6 2 1;1 5 6;8 4 3;3 7 8;6 7 3;3 2 6;5 1 4;4 8 5;4 1 2;2 3 4;7 6 5;5 8 7],'RCSPattern',[10 10;10 10],'RCSAzimuthAngles',[-180 180],'RCSElevationAngles',[-90 90]); struct('ActorID',4,'ClassID',1,'Length',4.7,'Width',1.8,'Height',1.4,'OriginOffset',[-1.35 0 0],'MeshVertices',[3.7 -0.9 1.4;3.7 0.9 1.4;-1 0.9 1.4;-1 -0.9 1.4;3.7 -0.9 0;3.7 0.9 0;-1 0.9 0;-1 -0.9 0],'MeshFaces',[6 2 1;1 5 6;8 4 3;3 7 8;6 7 3;3 2 6;5 1 4;4 8 5;4 1 2;2 3 4;7 6 5;5 8 7],'RCSPattern',[10 10;10 10],'RCSAzimuthAngles',[-180 180],'RCSElevationAngles',[-90 90]); struct('ActorID',5,'ClassID',1,'Length',4.7,'Width',1.8,'Height',1.4,'OriginOffset',[-1.35 0 0],'MeshVertices',[3.7 -0.9 1.4;3.7 0.9 1.4;-1 0.9 1.4;-1 -0.9 1.4;3.7 -0.9 0;3.7 0.9 0;-1 0.9 0;-1 -0.9 0],'MeshFaces',[6 2 1;1 5 6;8 4 3;3 7 8;6 7 3;3 2 6;5 1 4;4 8 5;4 1 2;2 3 4;7 6 5;5 8 7],'RCSPattern',[10 10;10 10],'RCSAzimuthAngles',[-180 180],'RCSElevationAngles',[-90 90]); struct('ActorID',6,'ClassID',4,'Length',0.24,'Width',0.45,'Height',1.7,'OriginOffset',[0 0 0],'MeshVertices',[0.12 -0.225 1.7;0.12 0.225 1.7;-0.12 0.225 1.7;-0.12 -0.225 1.7;0.12 -0.225 -1.11022302462516e-16;0.12 0.225 -1.11022302462516e-16;-0.12 0.225 -1.11022302462516e-16;-0.12 -0.225 -1.11022302462516e-16],'MeshFaces',[6 2 1;1 5 6;8 4 3;3 7 8;6 7 3;3 2 6;5 1 4;4 8 5;4 1 2;2 3 4;7 6 5;5 8 7],'RCSPattern',[-8 -8;-8 -8],'RCSAzimuthAngles',[-180 180],'RCSElevationAngles',[-90 90]); struct('ActorID',7,'ClassID',4,'Length',0.24,'Width',0.45,'Height',1.7,'OriginOffset',[0 0 0],'MeshVertices',[0.12 -0.225 1.7;0.12 0.225 1.7;-0.12 0.225 1.7;-0.12 -0.225 1.7;0.12 -0.225 -1.11022302462516e-16;0.12 0.225 -1.11022302462516e-16;-0.12 0.225 -1.11022302462516e-16;-0.12 -0.225 -1.11022302462516e-16],'MeshFaces',[6 2 1;1 5 6;8 4 3;3 7 8;6 7 3;3 2 6;5 1 4;4 8 5;4 1 2;2 3 4;7 6 5;5 8 7],'RCSPattern',[-8 -8;-8 -8],'RCSAzimuthAngles',[-180 180],'RCSElevationAngles',[-90 90]); struct('ActorID',8,'ClassID',4,'Length',0.24,'Width',0.45,'Height',1.7,'OriginOffset',[0 0 0],'MeshVertices',[0.12 -0.225 1.7;0.12 0.225 1.7;-0.12 0.225 1.7;-0.12 -0.225 1.7;0.12 -0.225 -1.11022302462516e-16;0.12 0.225 -1.11022302462516e-16;-0.12 0.225 -1.11022302462516e-16;-0.12 -0.225 -1.11022302462516e-16],'MeshFaces',[6 2 1;1 5 6;8 4 3;3 7 8;6 7 3;3 2 6;5 1 4;4 8 5;4 1 2;2 3 4;7 6 5;5 8 7],'RCSPattern',[-8 -8;-8 -8],'RCSAzimuthAngles',[-180 180],'RCSElevationAngles',[-90 90]); struct('ActorID',9,'ClassID',4,'Length',0.24,'Width',0.45,'Height',1.7,'OriginOffset',[0 0 0],'MeshVertices',[0.12 -0.225 1.7;0.12 0.225 1.7;-0.12 0.225 1.7;-0.12 -0.225 1.7;0.12 -0.225 -1.11022302462516e-16;0.12 0.225 -1.11022302462516e-16;-0.12 0.225 -1.11022302462516e-16;-0.12 -0.225 -1.11022302462516e-16],'MeshFaces',[6 2 1;1 5 6;8 4 3;3 7 8;6 7 3;3 2 6;5 1 4;4 8 5;4 1 2;2 3 4;7 6 5;5 8 7],'RCSPattern',[-8 -8;-8 -8],'RCSAzimuthAngles',[-180 180],'RCSElevationAngles',[-90 90]); struct('ActorID',10,'ClassID',4,'Length',0.24,'Width',0.45,'Height',1.7,'OriginOffset',[0 0 0],'MeshVertices',[0.12 -0.225 1.7;0.12 0.225 1.7;-0.12 0.225 1.7;-0.12 -0.225 1.7;0.12 -0.225 -1.11022302462516e-16;0.12 0.225 -1.11022302462516e-16;-0.12 0.225 -1.11022302462516e-16;-0.12 -0.225 -1.11022302462516e-16],'MeshFaces',[6 2 1;1 5 6;8 4 3;3 7 8;6 7 3;3 2 6;5 1 4;4 8 5;4 1 2;2 3 4;7 6 5;5 8 7],'RCSPattern',[-8 -8;-8 -8],'RCSAzimuthAngles',[-180 180],'RCSElevationAngles',[-90 90]); struct('ActorID',11,'ClassID',4,'Length',0.24,'Width',0.45,'Height',1.7,'OriginOffset',[0 0 0],'MeshVertices',[0.12 -0.225 1.7;0.12 0.225 1.7;-0.12 0.225 1.7;-0.12 -0.225 1.7;0.12 -0.225 -1.11022302462516e-16;0.12 0.225 -1.11022302462516e-16;-0.12 0.225 -1.11022302462516e-16;-0.12 -0.225 -1.11022302462516e-16],'MeshFaces',[6 2 1;1 5 6;8 4 3;3 7 8;6 7 3;3 2 6;5 1 4;4 8 5;4 1 2;2 3 4;7 6 5;5 8 7],'RCSPattern',[-8 -8;-8 -8],'RCSAzimuthAngles',[-180 180],'RCSElevationAngles',[-90 90]); struct('ActorID',12,'ClassID',4,'Length',0.24,'Width',0.45,'Height',1.7,'OriginOffset',[0 0 0],'MeshVertices',[0.12 -0.225 1.7;0.12 0.225 1.7;-0.12 0.225 1.7;-0.12 -0.225 1.7;0.12 -0.225 -1.11022302462516e-16;0.12 0.225 -1.11022302462516e-16;-0.12 0.225 -1.11022302462516e-16;-0.12 -0.225 -1.11022302462516e-16],'MeshFaces',[6 2 1;1 5 6;8 4 3;3 7 8;6 7 3;3 2 6;5 1 4;4 8 5;4 1 2;2 3 4;7 6 5;5 8 7],'RCSPattern',[-8 -8;-8 -8],'RCSAzimuthAngles',[-180 180],'RCSElevationAngles',[-90 90]); struct('ActorID',13,'ClassID',4,'Length',0.24,'Width',0.45,'Height',1.7,'OriginOffset',[0 0 0],'MeshVertices',[0.12 -0.225 1.7;0.12 0.225 1.7;-0.12 0.225 1.7;-0.12 -0.225 1.7;0.12 -0.225 -1.11022302462516e-16;0.12 0.225 -1.11022302462516e-16;-0.12 0.225 -1.11022302462516e-16;-0.12 -0.225 -1.11022302462516e-16],'MeshFaces',[6 2 1;1 5 6;8 4 3;3 7 8;6 7 3;3 2 6;5 1 4;4 8 5;4 1 2;2 3 4;7 6 5;5 8 7],'RCSPattern',[-8 -8;-8 -8],'RCSAzimuthAngles',[-180 180],'RCSElevationAngles',[-90 90]); struct('ActorID',14,'ClassID',4,'Length',0.24,'Width',0.45,'Height',1.7,'OriginOffset',[0 0 0],'MeshVertices',[0.12 -0.225 1.7;0.12 0.225 1.7;-0.12 0.225 1.7;-0.12 -0.225 1.7;0.12 -0.225 -1.11022302462516e-16;0.12 0.225 -1.11022302462516e-16;-0.12 0.225 -1.11022302462516e-16;-0.12 -0.225 -1.11022302462516e-16],'MeshFaces',[6 2 1;1 5 6;8 4 3;3 7 8;6 7 3;3 2 6;5 1 4;4 8 5;4 1 2;2 3 4;7 6 5;5 8 7],'RCSPattern',[-8 -8;-8 -8],'RCSAzimuthAngles',[-180 180],'RCSElevationAngles',[-90 90]); struct('ActorID',15,'ClassID',4,'Length',0.24,'Width',0.45,'Height',1.7,'OriginOffset',[0 0 0],'MeshVertices',[0.12 -0.225 1.7;0.12 0.225 1.7;-0.12 0.225 1.7;-0.12 -0.225 1.7;0.12 -0.225 -1.11022302462516e-16;0.12 0.225 -1.11022302462516e-16;-0.12 0.225 -1.11022302462516e-16;-0.12 -0.225 -1.11022302462516e-16],'MeshFaces',[6 2 1;1 5 6;8 4 3;3 7 8;6 7 3;3 2 6;5 1 4;4 8 5;4 1 2;2 3 4;7 6 5;5 8 7],'RCSPattern',[-8 -8;-8 -8],'RCSAzimuthAngles',[-180 180],'RCSElevationAngles',[-90 90]); struct('ActorID',16,'ClassID',4,'Length',0.24,'Width',0.45,'Height',1.7,'OriginOffset',[0 0 0],'MeshVertices',[0.12 -0.225 1.7;0.12 0.225 1.7;-0.12 0.225 1.7;-0.12 -0.225 1.7;0.12 -0.225 -1.11022302462516e-16;0.12 0.225 -1.11022302462516e-16;-0.12 0.225 -1.11022302462516e-16;-0.12 -0.225 -1.11022302462516e-16],'MeshFaces',[6 2 1;1 5 6;8 4 3;3 7 8;6 7 3;3 2 6;5 1 4;4 8 5;4 1 2;2 3 4;7 6 5;5 8 7],'RCSPattern',[-8 -8;-8 -8],'RCSAzimuthAngles',[-180 180],'RCSElevationAngles',[-90 90]); struct('ActorID',17,'ClassID',4,'Length',0.24,'Width',0.45,'Height',1.7,'OriginOffset',[0 0 0],'MeshVertices',[0.12 -0.225 1.7;0.12 0.225 1.7;-0.12 0.225 1.7;-0.12 -0.225 1.7;0.12 -0.225 -1.11022302462516e-16;0.12 0.225 -1.11022302462516e-16;-0.12 0.225 -1.11022302462516e-16;-0.12 -0.225 -1.11022302462516e-16],'MeshFaces',[6 2 1;1 5 6;8 4 3;3 7 8;6 7 3;3 2 6;5 1 4;4 8 5;4 1 2;2 3 4;7 6 5;5 8 7],'RCSPattern',[-8 -8;-8 -8],'RCSAzimuthAngles',[-180 180],'RCSElevationAngles',[-90 90]); struct('ActorID',18,'ClassID',4,'Length',0.24,'Width',0.45,'Height',1.7,'OriginOffset',[0 0 0],'MeshVertices',[0.12 -0.225 1.7;0.12 0.225 1.7;-0.12 0.225 1.7;-0.12 -0.225 1.7;0.12 -0.225 -1.11022302462516e-16;0.12 0.225 -1.11022302462516e-16;-0.12 0.225 -1.11022302462516e-16;-0.12 -0.225 -1.11022302462516e-16],'MeshFaces',[6 2 1;1 5 6;8 4 3;3 7 8;6 7 3;3 2 6;5 1 4;4 8 5;4 1 2;2 3 4;7 6 5;5 8 7],'RCSPattern',[-8 -8;-8 -8],'RCSAzimuthAngles',[-180 180],'RCSElevationAngles',[-90 90]); struct('ActorID',19,'ClassID',4,'Length',0.24,'Width',0.45,'Height',1.7,'OriginOffset',[0 0 0],'MeshVertices',[0.12 -0.225 1.7;0.12 0.225 1.7;-0.12 0.225 1.7;-0.12 -0.225 1.7;0.12 -0.225 -1.11022302462516e-16;0.12 0.225 -1.11022302462516e-16;-0.12 0.225 -1.11022302462516e-16;-0.12 -0.225 -1.11022302462516e-16],'MeshFaces',[6 2 1;1 5 6;8 4 3;3 7 8;6 7 3;3 2 6;5 1 4;4 8 5;4 1 2;2 3 4;7 6 5;5 8 7],'RCSPattern',[-8 -8;-8 -8],'RCSAzimuthAngles',[-180 180],'RCSElevationAngles',[-90 90]); struct('ActorID',20,'ClassID',4,'Length',0.24,'Width',0.45,'Height',1.7,'OriginOffset',[0 0 0],'MeshVertices',[0.12 -0.225 1.7;0.12 0.225 1.7;-0.12 0.225 1.7;-0.12 -0.225 1.7;0.12 -0.225 -1.11022302462516e-16;0.12 0.225 -1.11022302462516e-16;-0.12 0.225 -1.11022302462516e-16;-0.12 -0.225 -1.11022302462516e-16],'MeshFaces',[6 2 1;1 5 6;8 4 3;3 7 8;6 7 3;3 2 6;5 1 4;4 8 5;4 1 2;2 3 4;7 6 5;5 8 7],'RCSPattern',[-8 -8;-8 -8],'RCSAzimuthAngles',[-180 180],'RCSElevationAngles',[-90 90]); struct('ActorID',21,'ClassID',4,'Length',0.24,'Width',0.45,'Height',1.7,'OriginOffset',[0 0 0],'MeshVertices',[0.12 -0.225 1.7;0.12 0.225 1.7;-0.12 0.225 1.7;-0.12 -0.225 1.7;0.12 -0.225 -1.11022302462516e-16;0.12 0.225 -1.11022302462516e-16;-0.12 0.225 -1.11022302462516e-16;-0.12 -0.225 -1.11022302462516e-16],'MeshFaces',[6 2 1;1 5 6;8 4 3;3 7 8;6 7 3;3 2 6;5 1 4;4 8 5;4 1 2;2 3 4;7 6 5;5 8 7],'RCSPattern',[-8 -8;-8 -8],'RCSAzimuthAngles',[-180 180],'RCSElevationAngles',[-90 90]); struct('ActorID',22,'ClassID',4,'Length',0.24,'Width',0.45,'Height',1.7,'OriginOffset',[0 0 0],'MeshVertices',[0.12 -0.225 1.7;0.12 0.225 1.7;-0.12 0.225 1.7;-0.12 -0.225 1.7;0.12 -0.225 -1.11022302462516e-16;0.12 0.225 -1.11022302462516e-16;-0.12 0.225 -1.11022302462516e-16;-0.12 -0.225 -1.11022302462516e-16],'MeshFaces',[6 2 1;1 5 6;8 4 3;3 7 8;6 7 3;3 2 6;5 1 4;4 8 5;4 1 2;2 3 4;7 6 5;5 8 7],'RCSPattern',[-8 -8;-8 -8],'RCSAzimuthAngles',[-180 180],'RCSElevationAngles',[-90 90]); struct('ActorID',23,'ClassID',4,'Length',0.24,'Width',0.45,'Height',1.7,'OriginOffset',[0 0 0],'MeshVertices',[0.12 -0.225 1.7;0.12 0.225 1.7;-0.12 0.225 1.7;-0.12 -0.225 1.7;0.12 -0.225 -1.11022302462516e-16;0.12 0.225 -1.11022302462516e-16;-0.12 0.225 -1.11022302462516e-16;-0.12 -0.225 -1.11022302462516e-16],'MeshFaces',[6 2 1;1 5 6;8 4 3;3 7 8;6 7 3;3 2 6;5 1 4;4 8 5;4 1 2;2 3 4;7 6 5;5 8 7],'RCSPattern',[-8 -8;-8 -8],'RCSAzimuthAngles',[-180 180],'RCSElevationAngles',[-90 90]); struct('ActorID',24,'ClassID',4,'Length',0.24,'Width',0.45,'Height',1.7,'OriginOffset',[0 0 0],'MeshVertices',[0.12 -0.225 1.7;0.12 0.225 1.7;-0.12 0.225 1.7;-0.12 -0.225 1.7;0.12 -0.225 -1.11022302462516e-16;0.12 0.225 -1.11022302462516e-16;-0.12 0.225 -1.11022302462516e-16;-0.12 -0.225 -1.11022302462516e-16],'MeshFaces',[6 2 1;1 5 6;8 4 3;3 7 8;6 7 3;3 2 6;5 1 4;4 8 5;4 1 2;2 3 4;7 6 5;5 8 7],'RCSPattern',[-8 -8;-8 -8],'RCSAzimuthAngles',[-180 180],'RCSElevationAngles',[-90 90]); struct('ActorID',25,'ClassID',4,'Length',0.24,'Width',0.45,'Height',1.7,'OriginOffset',[0 0 0],'MeshVertices',[0.12 -0.225 1.7;0.12 0.225 1.7;-0.12 0.225 1.7;-0.12 -0.225 1.7;0.12 -0.225 -1.11022302462516e-16;0.12 0.225 -1.11022302462516e-16;-0.12 0.225 -1.11022302462516e-16;-0.12 -0.225 -1.11022302462516e-16],'MeshFaces',[6 2 1;1 5 6;8 4 3;3 7 8;6 7 3;3 2 6;5 1 4;4 8 5;4 1 2;2 3 4;7 6 5;5 8 7],'RCSPattern',[-8 -8;-8 -8],'RCSAzimuthAngles',[-180 180],'RCSElevationAngles',[-90 90]); struct('ActorID',26,'ClassID',4,'Length',0.24,'Width',0.45,'Height',1.7,'OriginOffset',[0 0 0],'MeshVertices',[0.12 -0.225 1.7;0.12 0.225 1.7;-0.12 0.225 1.7;-0.12 -0.225 1.7;0.12 -0.225 -1.11022302462516e-16;0.12 0.225 -1.11022302462516e-16;-0.12 0.225 -1.11022302462516e-16;-0.12 -0.225 -1.11022302462516e-16],'MeshFaces',[6 2 1;1 5 6;8 4 3;3 7 8;6 7 3;3 2 6;5 1 4;4 8 5;4 1 2;2 3 4;7 6 5;5 8 7],'RCSPattern',[-8 -8;-8 -8],'RCSAzimuthAngles',[-180 180],'RCSElevationAngles',[-90 90]); struct('ActorID',27,'ClassID',4,'Length',0.24,'Width',0.45,'Height',1.7,'OriginOffset',[0 0 0],'MeshVertices',[0.12 -0.225 1.7;0.12 0.225 1.7;-0.12 0.225 1.7;-0.12 -0.225 1.7;0.12 -0.225 -1.11022302462516e-16;0.12 0.225 -1.11022302462516e-16;-0.12 0.225 -1.11022302462516e-16;-0.12 -0.225 -1.11022302462516e-16],'MeshFaces',[6 2 1;1 5 6;8 4 3;3 7 8;6 7 3;3 2 6;5 1 4;4 8 5;4 1 2;2 3 4;7 6 5;5 8 7],'RCSPattern',[-8 -8;-8 -8],'RCSAzimuthAngles',[-180 180],'RCSElevationAngles',[-90 90]); struct('ActorID',28,'ClassID',3,'Length',1.7,'Width',0.45,'Height',1.7,'OriginOffset',[0 0 0],'MeshVertices',[0.85 -0.225 1.7;0.85 0.225 1.7;-0.85 0.225 1.7;-0.85 -0.225 1.7;0.85 -0.225 -1.11022302462516e-16;0.85 0.225 -1.11022302462516e-16;-0.85 0.225 -1.11022302462516e-16;-0.85 -0.225 -1.11022302462516e-16],'MeshFaces',[6 2 1;1 5 6;8 4 3;3 7 8;6 7 3;3 2 6;5 1 4;4 8 5;4 1 2;2 3 4;7 6 5;5 8 7],'RCSPattern',[10 10;10 10],'RCSAzimuthAngles',[-180 180],'RCSElevationAngles',[-90 90]); struct('ActorID',29,'ClassID',4,'Length',0.24,'Width',0.45,'Height',1.7,'OriginOffset',[0 0 0],'MeshVertices',[0.12 -0.225 1.7;0.12 0.225 1.7;-0.12 0.225 1.7;-0.12 -0.225 1.7;0.12 -0.225 -1.11022302462516e-16;0.12 0.225 -1.11022302462516e-16;-0.12 0.225 -1.11022302462516e-16;-0.12 -0.225 -1.11022302462516e-16],'MeshFaces',[6 2 1;1 5 6;8 4 3;3 7 8;6 7 3;3 2 6;5 1 4;4 8 5;4 1 2;2 3 4;7 6 5;5 8 7],'RCSPattern',[-8 -8;-8 -8],'RCSAzimuthAngles',[-180 180],'RCSElevationAngles',[-90 90])]
      settings: SourceProductBaseCode=DR
  Radar6 : drivingscenarioandsensors/Radar Detection Generator  SensorIndex=13  UpdateInterval=0.1  SensorLocation=[1.9 0]  Height=0.2  Yaw=-98.2594379798788  Pitch=0  Roll=0  BusNameSource=Auto  BusName=BusRadarDetectionGenerator  MaxNumDetectionsSource=Property  MaxNumDetections=50  DetectionCoordinates=Ego Cartesian  SimulateUsing=Interpreted execution  AzimuthResolution=4  ElevationResolution=10  RangeResolution=2.5  RangeRateResolution=0.5  AzimuthBiasFraction=0.1  ElevationBiasFraction=0.1  RangeBiasFraction=0.05  RangeRateBiasFraction=0.05  FieldOfView=[90 2.5]  MaxRange=10  RangeRateLimits=[-100 100]  DetectionProbability=0.9  FalseAlarmRate=1e-06  ReferenceRange=15  ReferenceRCS=0  HasElevation=on  HasRangeRate=off  HasNoise=on  HasFalseAlarms=on  HasOcclusion=on  InitialSeedSource=Repeatable  InitialSeed=0  UsedSeed=0  ActorProfilesSource=MATLAB expression  ActorProfilesParameters=driving.internal.ActorProfilesRadarParameters  ActorProfilesExpression=[struct('ActorID',1,'ClassID',1,'Length',4.7,'Width',1.8,'Height',1.4,'OriginOffset',[-1.35 0 0],'MeshVertices',[3.7 -0.9 1.4;3.7 0.9 1.4;-1 0.9 1.4;-1 -0.9 1.4;3.7 -0.9 0;3.7 0.9 0;-1 0.9 0;-1 -0.9 0],'MeshFaces',[6 2 1;1 5 6;8 4 3;3 7 8;6 7 3;3 2 6;5 1 4;4 8 5;4 1 2;2 3 4;7 6 5;5 8 7],'RCSPattern',[10 10;10 10],'RCSAzimuthAngles',[-180 180],'RCSElevationAngles',[-90 90]); struct('ActorID',2,'ClassID',1,'Length',4.7,'Width',1.8,'Height',1.4,'OriginOffset',[-1.35 0 0],'MeshVertices',[3.7 -0.9 1.4;3.7 0.9 1.4;-1 0.9 1.4;-1 -0.9 1.4;3.7 -0.9 0;3.7 0.9 0;-1 0.9 0;-1 -0.9 0],'MeshFaces',[6 2 1;1 5 6;8 4 3;3 7 8;6 7 3;3 2 6;5 1 4;4 8 5;4 1 2;2 3 4;7 6 5;5 8 7],'RCSPattern',[10 10;10 10],'RCSAzimuthAngles',[-180 180],'RCSElevationAngles',[-90 90]); struct('ActorID',3,'ClassID',1,'Length',4.7,'Width',1.8,'Height',1.4,'OriginOffset',[-1.35 0 0],'MeshVertices',[3.7 -0.9 1.4;3.7 0.9 1.4;-1 0.9 1.4;-1 -0.9 1.4;3.7 -0.9 0;3.7 0.9 0;-1 0.9 0;-1 -0.9 0],'MeshFaces',[6 2 1;1 5 6;8 4 3;3 7 8;6 7 3;3 2 6;5 1 4;4 8 5;4 1 2;2 3 4;7 6 5;5 8 7],'RCSPattern',[10 10;10 10],'RCSAzimuthAngles',[-180 180],'RCSElevationAngles',[-90 90]); struct('ActorID',4,'ClassID',1,'Length',4.7,'Width',1.8,'Height',1.4,'OriginOffset',[-1.35 0 0],'MeshVertices',[3.7 -0.9 1.4;3.7 0.9 1.4;-1 0.9 1.4;-1 -0.9 1.4;3.7 -0.9 0;3.7 0.9 0;-1 0.9 0;-1 -0.9 0],'MeshFaces',[6 2 1;1 5 6;8 4 3;3 7 8;6 7 3;3 2 6;5 1 4;4 8 5;4 1 2;2 3 4;7 6 5;5 8 7],'RCSPattern',[10 10;10 10],'RCSAzimuthAngles',[-180 180],'RCSElevationAngles',[-90 90]); struct('ActorID',5,'ClassID',1,'Length',4.7,'Width',1.8,'Height',1.4,'OriginOffset',[-1.35 0 0],'MeshVertices',[3.7 -0.9 1.4;3.7 0.9 1.4;-1 0.9 1.4;-1 -0.9 1.4;3.7 -0.9 0;3.7 0.9 0;-1 0.9 0;-1 -0.9 0],'MeshFaces',[6 2 1;1 5 6;8 4 3;3 7 8;6 7 3;3 2 6;5 1 4;4 8 5;4 1 2;2 3 4;7 6 5;5 8 7],'RCSPattern',[10 10;10 10],'RCSAzimuthAngles',[-180 180],'RCSElevationAngles',[-90 90]); struct('ActorID',6,'ClassID',4,'Length',0.24,'Width',0.45,'Height',1.7,'OriginOffset',[0 0 0],'MeshVertices',[0.12 -0.225 1.7;0.12 0.225 1.7;-0.12 0.225 1.7;-0.12 -0.225 1.7;0.12 -0.225 -1.11022302462516e-16;0.12 0.225 -1.11022302462516e-16;-0.12 0.225 -1.11022302462516e-16;-0.12 -0.225 -1.11022302462516e-16],'MeshFaces',[6 2 1;1 5 6;8 4 3;3 7 8;6 7 3;3 2 6;5 1 4;4 8 5;4 1 2;2 3 4;7 6 5;5 8 7],'RCSPattern',[-8 -8;-8 -8],'RCSAzimuthAngles',[-180 180],'RCSElevationAngles',[-90 90]); struct('ActorID',7,'ClassID',4,'Length',0.24,'Width',0.45,'Height',1.7,'OriginOffset',[0 0 0],'MeshVertices',[0.12 -0.225 1.7;0.12 0.225 1.7;-0.12 0.225 1.7;-0.12 -0.225 1.7;0.12 -0.225 -1.11022302462516e-16;0.12 0.225 -1.11022302462516e-16;-0.12 0.225 -1.11022302462516e-16;-0.12 -0.225 -1.11022302462516e-16],'MeshFaces',[6 2 1;1 5 6;8 4 3;3 7 8;6 7 3;3 2 6;5 1 4;4 8 5;4 1 2;2 3 4;7 6 5;5 8 7],'RCSPattern',[-8 -8;-8 -8],'RCSAzimuthAngles',[-180 180],'RCSElevationAngles',[-90 90]); struct('ActorID',8,'ClassID',4,'Length',0.24,'Width',0.45,'Height',1.7,'OriginOffset',[0 0 0],'MeshVertices',[0.12 -0.225 1.7;0.12 0.225 1.7;-0.12 0.225 1.7;-0.12 -0.225 1.7;0.12 -0.225 -1.11022302462516e-16;0.12 0.225 -1.11022302462516e-16;-0.12 0.225 -1.11022302462516e-16;-0.12 -0.225 -1.11022302462516e-16],'MeshFaces',[6 2 1;1 5 6;8 4 3;3 7 8;6 7 3;3 2 6;5 1 4;4 8 5;4 1 2;2 3 4;7 6 5;5 8 7],'RCSPattern',[-8 -8;-8 -8],'RCSAzimuthAngles',[-180 180],'RCSElevationAngles',[-90 90]); struct('ActorID',9,'ClassID',4,'Length',0.24,'Width',0.45,'Height',1.7,'OriginOffset',[0 0 0],'MeshVertices',[0.12 -0.225 1.7;0.12 0.225 1.7;-0.12 0.225 1.7;-0.12 -0.225 1.7;0.12 -0.225 -1.11022302462516e-16;0.12 0.225 -1.11022302462516e-16;-0.12 0.225 -1.11022302462516e-16;-0.12 -0.225 -1.11022302462516e-16],'MeshFaces',[6 2 1;1 5 6;8 4 3;3 7 8;6 7 3;3 2 6;5 1 4;4 8 5;4 1 2;2 3 4;7 6 5;5 8 7],'RCSPattern',[-8 -8;-8 -8],'RCSAzimuthAngles',[-180 180],'RCSElevationAngles',[-90 90]); struct('ActorID',10,'ClassID',4,'Length',0.24,'Width',0.45,'Height',1.7,'OriginOffset',[0 0 0],'MeshVertices',[0.12 -0.225 1.7;0.12 0.225 1.7;-0.12 0.225 1.7;-0.12 -0.225 1.7;0.12 -0.225 -1.11022302462516e-16;0.12 0.225 -1.11022302462516e-16;-0.12 0.225 -1.11022302462516e-16;-0.12 -0.225 -1.11022302462516e-16],'MeshFaces',[6 2 1;1 5 6;8 4 3;3 7 8;6 7 3;3 2 6;5 1 4;4 8 5;4 1 2;2 3 4;7 6 5;5 8 7],'RCSPattern',[-8 -8;-8 -8],'RCSAzimuthAngles',[-180 180],'RCSElevationAngles',[-90 90]); struct('ActorID',11,'ClassID',4,'Length',0.24,'Width',0.45,'Height',1.7,'OriginOffset',[0 0 0],'MeshVertices',[0.12 -0.225 1.7;0.12 0.225 1.7;-0.12 0.225 1.7;-0.12 -0.225 1.7;0.12 -0.225 -1.11022302462516e-16;0.12 0.225 -1.11022302462516e-16;-0.12 0.225 -1.11022302462516e-16;-0.12 -0.225 -1.11022302462516e-16],'MeshFaces',[6 2 1;1 5 6;8 4 3;3 7 8;6 7 3;3 2 6;5 1 4;4 8 5;4 1 2;2 3 4;7 6 5;5 8 7],'RCSPattern',[-8 -8;-8 -8],'RCSAzimuthAngles',[-180 180],'RCSElevationAngles',[-90 90]); struct('ActorID',12,'ClassID',4,'Length',0.24,'Width',0.45,'Height',1.7,'OriginOffset',[0 0 0],'MeshVertices',[0.12 -0.225 1.7;0.12 0.225 1.7;-0.12 0.225 1.7;-0.12 -0.225 1.7;0.12 -0.225 -1.11022302462516e-16;0.12 0.225 -1.11022302462516e-16;-0.12 0.225 -1.11022302462516e-16;-0.12 -0.225 -1.11022302462516e-16],'MeshFaces',[6 2 1;1 5 6;8 4 3;3 7 8;6 7 3;3 2 6;5 1 4;4 8 5;4 1 2;2 3 4;7 6 5;5 8 7],'RCSPattern',[-8 -8;-8 -8],'RCSAzimuthAngles',[-180 180],'RCSElevationAngles',[-90 90]); struct('ActorID',13,'ClassID',4,'Length',0.24,'Width',0.45,'Height',1.7,'OriginOffset',[0 0 0],'MeshVertices',[0.12 -0.225 1.7;0.12 0.225 1.7;-0.12 0.225 1.7;-0.12 -0.225 1.7;0.12 -0.225 -1.11022302462516e-16;0.12 0.225 -1.11022302462516e-16;-0.12 0.225 -1.11022302462516e-16;-0.12 -0.225 -1.11022302462516e-16],'MeshFaces',[6 2 1;1 5 6;8 4 3;3 7 8;6 7 3;3 2 6;5 1 4;4 8 5;4 1 2;2 3 4;7 6 5;5 8 7],'RCSPattern',[-8 -8;-8 -8],'RCSAzimuthAngles',[-180 180],'RCSElevationAngles',[-90 90]); struct('ActorID',14,'ClassID',4,'Length',0.24,'Width',0.45,'Height',1.7,'OriginOffset',[0 0 0],'MeshVertices',[0.12 -0.225 1.7;0.12 0.225 1.7;-0.12 0.225 1.7;-0.12 -0.225 1.7;0.12 -0.225 -1.11022302462516e-16;0.12 0.225 -1.11022302462516e-16;-0.12 0.225 -1.11022302462516e-16;-0.12 -0.225 -1.11022302462516e-16],'MeshFaces',[6 2 1;1 5 6;8 4 3;3 7 8;6 7 3;3 2 6;5 1 4;4 8 5;4 1 2;2 3 4;7 6 5;5 8 7],'RCSPattern',[-8 -8;-8 -8],'RCSAzimuthAngles',[-180 180],'RCSElevationAngles',[-90 90]); struct('ActorID',15,'ClassID',4,'Length',0.24,'Width',0.45,'Height',1.7,'OriginOffset',[0 0 0],'MeshVertices',[0.12 -0.225 1.7;0.12 0.225 1.7;-0.12 0.225 1.7;-0.12 -0.225 1.7;0.12 -0.225 -1.11022302462516e-16;0.12 0.225 -1.11022302462516e-16;-0.12 0.225 -1.11022302462516e-16;-0.12 -0.225 -1.11022302462516e-16],'MeshFaces',[6 2 1;1 5 6;8 4 3;3 7 8;6 7 3;3 2 6;5 1 4;4 8 5;4 1 2;2 3 4;7 6 5;5 8 7],'RCSPattern',[-8 -8;-8 -8],'RCSAzimuthAngles',[-180 180],'RCSElevationAngles',[-90 90]); struct('ActorID',16,'ClassID',4,'Length',0.24,'Width',0.45,'Height',1.7,'OriginOffset',[0 0 0],'MeshVertices',[0.12 -0.225 1.7;0.12 0.225 1.7;-0.12 0.225 1.7;-0.12 -0.225 1.7;0.12 -0.225 -1.11022302462516e-16;0.12 0.225 -1.11022302462516e-16;-0.12 0.225 -1.11022302462516e-16;-0.12 -0.225 -1.11022302462516e-16],'MeshFaces',[6 2 1;1 5 6;8 4 3;3 7 8;6 7 3;3 2 6;5 1 4;4 8 5;4 1 2;2 3 4;7 6 5;5 8 7],'RCSPattern',[-8 -8;-8 -8],'RCSAzimuthAngles',[-180 180],'RCSElevationAngles',[-90 90]); struct('ActorID',17,'ClassID',4,'Length',0.24,'Width',0.45,'Height',1.7,'OriginOffset',[0 0 0],'MeshVertices',[0.12 -0.225 1.7;0.12 0.225 1.7;-0.12 0.225 1.7;-0.12 -0.225 1.7;0.12 -0.225 -1.11022302462516e-16;0.12 0.225 -1.11022302462516e-16;-0.12 0.225 -1.11022302462516e-16;-0.12 -0.225 -1.11022302462516e-16],'MeshFaces',[6 2 1;1 5 6;8 4 3;3 7 8;6 7 3;3 2 6;5 1 4;4 8 5;4 1 2;2 3 4;7 6 5;5 8 7],'RCSPattern',[-8 -8;-8 -8],'RCSAzimuthAngles',[-180 180],'RCSElevationAngles',[-90 90]); struct('ActorID',18,'ClassID',4,'Length',0.24,'Width',0.45,'Height',1.7,'OriginOffset',[0 0 0],'MeshVertices',[0.12 -0.225 1.7;0.12 0.225 1.7;-0.12 0.225 1.7;-0.12 -0.225 1.7;0.12 -0.225 -1.11022302462516e-16;0.12 0.225 -1.11022302462516e-16;-0.12 0.225 -1.11022302462516e-16;-0.12 -0.225 -1.11022302462516e-16],'MeshFaces',[6 2 1;1 5 6;8 4 3;3 7 8;6 7 3;3 2 6;5 1 4;4 8 5;4 1 2;2 3 4;7 6 5;5 8 7],'RCSPattern',[-8 -8;-8 -8],'RCSAzimuthAngles',[-180 180],'RCSElevationAngles',[-90 90]); struct('ActorID',19,'ClassID',4,'Length',0.24,'Width',0.45,'Height',1.7,'OriginOffset',[0 0 0],'MeshVertices',[0.12 -0.225 1.7;0.12 0.225 1.7;-0.12 0.225 1.7;-0.12 -0.225 1.7;0.12 -0.225 -1.11022302462516e-16;0.12 0.225 -1.11022302462516e-16;-0.12 0.225 -1.11022302462516e-16;-0.12 -0.225 -1.11022302462516e-16],'MeshFaces',[6 2 1;1 5 6;8 4 3;3 7 8;6 7 3;3 2 6;5 1 4;4 8 5;4 1 2;2 3 4;7 6 5;5 8 7],'RCSPattern',[-8 -8;-8 -8],'RCSAzimuthAngles',[-180 180],'RCSElevationAngles',[-90 90]); struct('ActorID',20,'ClassID',4,'Length',0.24,'Width',0.45,'Height',1.7,'OriginOffset',[0 0 0],'MeshVertices',[0.12 -0.225 1.7;0.12 0.225 1.7;-0.12 0.225 1.7;-0.12 -0.225 1.7;0.12 -0.225 -1.11022302462516e-16;0.12 0.225 -1.11022302462516e-16;-0.12 0.225 -1.11022302462516e-16;-0.12 -0.225 -1.11022302462516e-16],'MeshFaces',[6 2 1;1 5 6;8 4 3;3 7 8;6 7 3;3 2 6;5 1 4;4 8 5;4 1 2;2 3 4;7 6 5;5 8 7],'RCSPattern',[-8 -8;-8 -8],'RCSAzimuthAngles',[-180 180],'RCSElevationAngles',[-90 90]); struct('ActorID',21,'ClassID',4,'Length',0.24,'Width',0.45,'Height',1.7,'OriginOffset',[0 0 0],'MeshVertices',[0.12 -0.225 1.7;0.12 0.225 1.7;-0.12 0.225 1.7;-0.12 -0.225 1.7;0.12 -0.225 -1.11022302462516e-16;0.12 0.225 -1.11022302462516e-16;-0.12 0.225 -1.11022302462516e-16;-0.12 -0.225 -1.11022302462516e-16],'MeshFaces',[6 2 1;1 5 6;8 4 3;3 7 8;6 7 3;3 2 6;5 1 4;4 8 5;4 1 2;2 3 4;7 6 5;5 8 7],'RCSPattern',[-8 -8;-8 -8],'RCSAzimuthAngles',[-180 180],'RCSElevationAngles',[-90 90]); struct('ActorID',22,'ClassID',4,'Length',0.24,'Width',0.45,'Height',1.7,'OriginOffset',[0 0 0],'MeshVertices',[0.12 -0.225 1.7;0.12 0.225 1.7;-0.12 0.225 1.7;-0.12 -0.225 1.7;0.12 -0.225 -1.11022302462516e-16;0.12 0.225 -1.11022302462516e-16;-0.12 0.225 -1.11022302462516e-16;-0.12 -0.225 -1.11022302462516e-16],'MeshFaces',[6 2 1;1 5 6;8 4 3;3 7 8;6 7 3;3 2 6;5 1 4;4 8 5;4 1 2;2 3 4;7 6 5;5 8 7],'RCSPattern',[-8 -8;-8 -8],'RCSAzimuthAngles',[-180 180],'RCSElevationAngles',[-90 90]); struct('ActorID',23,'ClassID',4,'Length',0.24,'Width',0.45,'Height',1.7,'OriginOffset',[0 0 0],'MeshVertices',[0.12 -0.225 1.7;0.12 0.225 1.7;-0.12 0.225 1.7;-0.12 -0.225 1.7;0.12 -0.225 -1.11022302462516e-16;0.12 0.225 -1.11022302462516e-16;-0.12 0.225 -1.11022302462516e-16;-0.12 -0.225 -1.11022302462516e-16],'MeshFaces',[6 2 1;1 5 6;8 4 3;3 7 8;6 7 3;3 2 6;5 1 4;4 8 5;4 1 2;2 3 4;7 6 5;5 8 7],'RCSPattern',[-8 -8;-8 -8],'RCSAzimuthAngles',[-180 180],'RCSElevationAngles',[-90 90]); struct('ActorID',24,'ClassID',4,'Length',0.24,'Width',0.45,'Height',1.7,'OriginOffset',[0 0 0],'MeshVertices',[0.12 -0.225 1.7;0.12 0.225 1.7;-0.12 0.225 1.7;-0.12 -0.225 1.7;0.12 -0.225 -1.11022302462516e-16;0.12 0.225 -1.11022302462516e-16;-0.12 0.225 -1.11022302462516e-16;-0.12 -0.225 -1.11022302462516e-16],'MeshFaces',[6 2 1;1 5 6;8 4 3;3 7 8;6 7 3;3 2 6;5 1 4;4 8 5;4 1 2;2 3 4;7 6 5;5 8 7],'RCSPattern',[-8 -8;-8 -8],'RCSAzimuthAngles',[-180 180],'RCSElevationAngles',[-90 90]); struct('ActorID',25,'ClassID',4,'Length',0.24,'Width',0.45,'Height',1.7,'OriginOffset',[0 0 0],'MeshVertices',[0.12 -0.225 1.7;0.12 0.225 1.7;-0.12 0.225 1.7;-0.12 -0.225 1.7;0.12 -0.225 -1.11022302462516e-16;0.12 0.225 -1.11022302462516e-16;-0.12 0.225 -1.11022302462516e-16;-0.12 -0.225 -1.11022302462516e-16],'MeshFaces',[6 2 1;1 5 6;8 4 3;3 7 8;6 7 3;3 2 6;5 1 4;4 8 5;4 1 2;2 3 4;7 6 5;5 8 7],'RCSPattern',[-8 -8;-8 -8],'RCSAzimuthAngles',[-180 180],'RCSElevationAngles',[-90 90]); struct('ActorID',26,'ClassID',4,'Length',0.24,'Width',0.45,'Height',1.7,'OriginOffset',[0 0 0],'MeshVertices',[0.12 -0.225 1.7;0.12 0.225 1.7;-0.12 0.225 1.7;-0.12 -0.225 1.7;0.12 -0.225 -1.11022302462516e-16;0.12 0.225 -1.11022302462516e-16;-0.12 0.225 -1.11022302462516e-16;-0.12 -0.225 -1.11022302462516e-16],'MeshFaces',[6 2 1;1 5 6;8 4 3;3 7 8;6 7 3;3 2 6;5 1 4;4 8 5;4 1 2;2 3 4;7 6 5;5 8 7],'RCSPattern',[-8 -8;-8 -8],'RCSAzimuthAngles',[-180 180],'RCSElevationAngles',[-90 90]); struct('ActorID',27,'ClassID',4,'Length',0.24,'Width',0.45,'Height',1.7,'OriginOffset',[0 0 0],'MeshVertices',[0.12 -0.225 1.7;0.12 0.225 1.7;-0.12 0.225 1.7;-0.12 -0.225 1.7;0.12 -0.225 -1.11022302462516e-16;0.12 0.225 -1.11022302462516e-16;-0.12 0.225 -1.11022302462516e-16;-0.12 -0.225 -1.11022302462516e-16],'MeshFaces',[6 2 1;1 5 6;8 4 3;3 7 8;6 7 3;3 2 6;5 1 4;4 8 5;4 1 2;2 3 4;7 6 5;5 8 7],'RCSPattern',[-8 -8;-8 -8],'RCSAzimuthAngles',[-180 180],'RCSElevationAngles',[-90 90]); struct('ActorID',28,'ClassID',3,'Length',1.7,'Width',0.45,'Height',1.7,'OriginOffset',[0 0 0],'MeshVertices',[0.85 -0.225 1.7;0.85 0.225 1.7;-0.85 0.225 1.7;-0.85 -0.225 1.7;0.85 -0.225 -1.11022302462516e-16;0.85 0.225 -1.11022302462516e-16;-0.85 0.225 -1.11022302462516e-16;-0.85 -0.225 -1.11022302462516e-16],'MeshFaces',[6 2 1;1 5 6;8 4 3;3 7 8;6 7 3;3 2 6;5 1 4;4 8 5;4 1 2;2 3 4;7 6 5;5 8 7],'RCSPattern',[10 10;10 10],'RCSAzimuthAngles',[-180 180],'RCSElevationAngles',[-90 90]); struct('ActorID',29,'ClassID',4,'Length',0.24,'Width',0.45,'Height',1.7,'OriginOffset',[0 0 0],'MeshVertices',[0.12 -0.225 1.7;0.12 0.225 1.7;-0.12 0.225 1.7;-0.12 -0.225 1.7;0.12 -0.225 -1.11022302462516e-16;0.12 0.225 -1.11022302462516e-16;-0.12 0.225 -1.11022302462516e-16;-0.12 -0.225 -1.11022302462516e-16],'MeshFaces',[6 2 1;1 5 6;8 4 3;3 7 8;6 7 3;3 2 6;5 1 4;4 8 5;4 1 2;2 3 4;7 6 5;5 8 7],'RCSPattern',[-8 -8;-8 -8],'RCSAzimuthAngles',[-180 180],'RCSElevationAngles',[-90 90])]
      settings: SourceProductBaseCode=DR
  Camera Object Detections : Outport
  Radar Object Detections : Outport  Port=2
  Radar1 Object Detections : Outport  Port=3
  Radar2 Object Detections : Outport  Port=4
  Radar3 Object Detections : Outport  Port=5
  Radar4 Object Detections : Outport  Port=6
  Camera1 Object Detections : Outport  Port=7
  Camera2 Object Detections : Outport  Port=8
  Camera3 Object Detections : Outport  Port=9
  Camera4 Object Detections : Outport  Port=10
  Camera5 Object Detections : Outport  Port=11
  Radar5 Object Detections : Outport  Port=12
  Radar6 Object Detections : Outport  Port=13
  wires:
  Radar5/1 -> Radar5 Object Detections/1
  Camera1/1 -> Camera1 Object Detections/1
  Radar3/1 -> Radar3 Object Detections/1
  Radar4/1 -> Radar4 Object Detections/1
  Camera/1 -> Camera Object Detections/1
  Camera5/1 -> Camera5 Object Detections/1
  Actors/1 -> Radar6/1, Radar5/1, Camera5/1, Camera4/1, Camera3/1, Camera2/1, Camera1/1, Radar4/1, Radar3/1, Radar2/1, Radar1/1, Radar/1, Camera/1
  Camera2/1 -> Camera2 Object Detections/1
  Radar6/1 -> Radar6 Object Detections/1
  Camera3/1 -> Camera3 Object Detections/1
  Radar1/1 -> Radar1 Object Detections/1
  Radar2/1 -> Radar2 Object Detections/1
  Radar/1 -> Radar Object Detections/1
  Camera4/1 -> Camera4 Object Detections/1
